simulink model "PWMGenerator"  (R2025a)
settings: Solver=VariableStepAuto  StartTime=0.0  StopTime=10.0  RelTol=1e-3
libraries: simulink x1
settings Model: Creator=mahij  LastModifiedBy=mahij

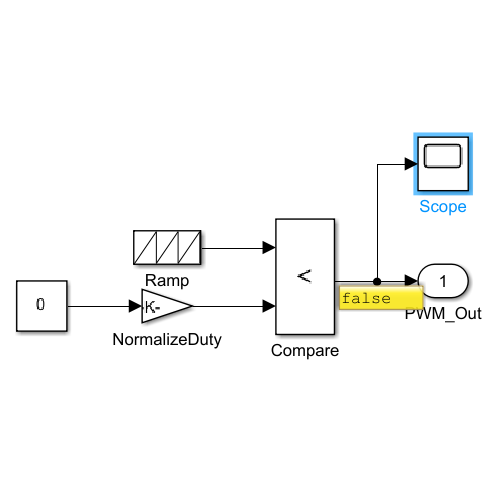
[thumbnail: Simulink's stored preview of the top-level diagram]
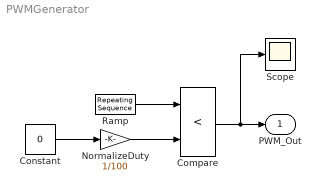
== system PWMGenerator ==
  Compare : RelationalOperator  Operator=<  OutDataTypeStr=boolean  RndMeth=Simplest  InputSameDT=off
  Constant : Constant  Value=0
  NormalizeDuty : Gain  Gain=1/100
  Ramp : simulink/Sources/Repeating Sequence  rep_seq_t=[0 0.001]  rep_seq_y=[0 1]
  Scope : Scope
      settings: ActiveDisplayYMinimum=-2.3630736714975846  ActiveDisplayYMaximum=2.6369263285024154
  PWM_Out : Outport
  wires:
  Constant/1 -> NormalizeDuty/1
  NormalizeDuty/1 -> Compare/2
  Ramp/1 -> Compare/1
  Compare/1 -> Scope/1, PWM_Out/1
